simulink model "Template"  (Simulink 7.3)
settings: Solver=ode45  StartTime=0.0  StopTime=10.0  RelTol=1e-3
undefined symbols (not defined in the file): eta1_0_real, v1_0_real, velocitySatValues1
libraries: dspmtrx3 x21, simulink x14, dspindex x5, marine_gnc x4, simulink_extras x1, dspinverses x1
(part 4 of 4)

== system Template/Main Subsystems/Guidance/Line-Of-Sight Path-Following/Path/Straight path/|p_d^s| eq ==
  p_d^s : Inport
  Product : Product  Multiplication=Matrix(*)  OutDataType=fixdt(1, 16)  OutScaling=2^0  RndMeth=Zero
  p_d^s^T : dspmtrx3/Transpose  SystemSampleTime=-1  Hermitian=off  overflowFlag=off
  sqrt : Math  Operator=sqrt  OutDataType=fixdt(1, 16)  OutScaling=2^0  SaturateOnIntegerOverflow=on
  |p_d^s| : Outport
  wires:
  p_d^s/1 -> Product/2, p_d^s^T/1
  sqrt/1 -> |p_d^s|/1
  Product/1 -> sqrt/1
  p_d^s^T/1 -> Product/1

== system Template/Main Subsystems/Guidance/Line-Of-Sight Path-Following/Line-Of-Sight/LOS heading/psi_los eq/rad to [-pi pi] ==
  rad : Inport  OutDataType=sfix(16)  OutScaling=2^0
  Constant : Constant  Value=2*pi  OutDataType=sfix(16)  OutScaling=2^0
  Gain : Gain  Gain=pi  ParameterDataType=sfix(16)  ParameterScaling=2^0  OutDataType=sfix(16)  OutScaling=2^0  SaturateOnIntegerOverflow=on  OutDataTypeStr=Inherit: Same as input  ParamDataTypeStr=Inherit: Same as input
  Math Function : Math  Operator=rem  OutDataType=sfix(16)  OutScaling=2^0  SaturateOnIntegerOverflow=on
  Saturation : Saturate  UpperLimit=1e10  LowerLimit=-1e10
  Sign : Signum
  Sum : Sum  Inputs=|+-  OutDataType=sfix(16)  OutScaling=2^0  SaturateOnIntegerOverflow=on
  Sum1 : Sum  Inputs=|++  OutDataType=sfix(16)  OutScaling=2^0  SaturateOnIntegerOverflow=on
  "[-pi pi]" : Outport  OutDataType=sfix(16)  OutScaling=2^0
  wires:
  Sum/1 -> "[-pi pi]"/1
  Math Function/1 -> Sum/1
  Constant/1 -> Math Function/2
  Sum1/1 -> Math Function/1
  Gain/1 -> Sum1/2, Sum/2
  Sign/1 -> Gain/1
  rad/1 -> Saturation/1
  Saturation/1 -> Sign/1, Sum1/1

== system Template/Main Subsystems/Guidance/Line-Of-Sight Path-Following/Line-Of-Sight/LOS heading/psi_los eq/rad to [-pi pi]1 ==
  rad : Inport  OutDataType=sfix(16)  OutScaling=2^0
  Constant : Constant  Value=2*pi  OutDataType=sfix(16)  OutScaling=2^0
  Gain : Gain  Gain=pi  ParameterDataType=sfix(16)  ParameterScaling=2^0  OutDataType=sfix(16)  OutScaling=2^0  SaturateOnIntegerOverflow=on  OutDataTypeStr=Inherit: Same as input  ParamDataTypeStr=Inherit: Same as input
  Math Function : Math  Operator=rem  OutDataType=sfix(16)  OutScaling=2^0  SaturateOnIntegerOverflow=on
  Saturation : Saturate  UpperLimit=1e10  LowerLimit=-1e10
  Sign : Signum
  Sum : Sum  Inputs=|+-  OutDataType=sfix(16)  OutScaling=2^0  SaturateOnIntegerOverflow=on
  Sum1 : Sum  Inputs=|++  OutDataType=sfix(16)  OutScaling=2^0  SaturateOnIntegerOverflow=on
  "[-pi pi]" : Outport  OutDataType=sfix(16)  OutScaling=2^0
  wires:
  Saturation/1 -> Sum1/1, Sign/1
  rad/1 -> Saturation/1
  Sign/1 -> Gain/1
  Gain/1 -> Sum/2, Sum1/2
  Sum1/1 -> Math Function/1
  Constant/1 -> Math Function/2
  Math Function/1 -> Sum/1
  Sum/1 -> "[-pi pi]"/1

== system Template/Main Subsystems/Guidance/Line-Of-Sight Path-Following/Line-Of-Sight/LOS heading/psi_los eq/rad to [-pi pi]2 ==
  rad : Inport  OutDataType=sfix(16)  OutScaling=2^0
  Constant : Constant  Value=2*pi  OutDataType=sfix(16)  OutScaling=2^0
  Gain : Gain  Gain=pi  ParameterDataType=sfix(16)  ParameterScaling=2^0  OutDataType=sfix(16)  OutScaling=2^0  SaturateOnIntegerOverflow=on  OutDataTypeStr=Inherit: Same as input  ParamDataTypeStr=Inherit: Same as input
  Math Function : Math  Operator=rem  OutDataType=sfix(16)  OutScaling=2^0  SaturateOnIntegerOverflow=on
  Saturation : Saturate  UpperLimit=1e10  LowerLimit=-1e10
  Sign : Signum
  Sum : Sum  Inputs=|+-  OutDataType=sfix(16)  OutScaling=2^0  SaturateOnIntegerOverflow=on
  Sum1 : Sum  Inputs=|++  OutDataType=sfix(16)  OutScaling=2^0  SaturateOnIntegerOverflow=on
  "[-pi pi]" : Outport  OutDataType=sfix(16)  OutScaling=2^0
  wires:
  Sum/1 -> "[-pi pi]"/1
  Math Function/1 -> Sum/1
  Constant/1 -> Math Function/2
  Sum1/1 -> Math Function/1
  Gain/1 -> Sum1/2, Sum/2
  Sign/1 -> Gain/1
  rad/1 -> Saturation/1
  Saturation/1 -> Sign/1, Sum1/1
